simulink model "HEncoder"  (R2018b)
settings: Solver=VariableStepAuto  StartTime=0.0  StopTime=10.0  RelTol=1e-3
settings Model: Creator=bai  LastModifiedBy=bai

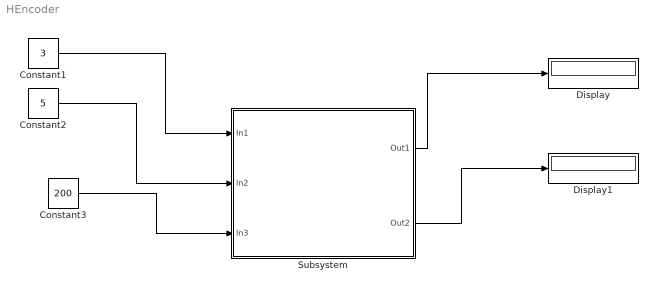
== system HEncoder ==
  Constant1 : Constant  Value=3
  Constant2 : Constant  Value=5
  Constant3 : Constant  Value=200
  Display : Display
  Display1 : Display
  Subsystem : Subsystem
      mask Display:
      | image('halleffect.jpg');
      | port_label('input', 1, 'A');
      | port_label('input', 2, 'B');
      | port_label('input', 3, 'sampleTIME');
      | port_label('output', 1, 'counter');
      | port_label('output', 2, 'rpm');
  wires:
  Constant1/1 -> Subsystem/1(In1)
  Constant2/1 -> Subsystem/2(In2)
  Constant3/1 -> Subsystem/3(In3)
  Subsystem/1(Out1) -> Display/1
  Subsystem/2(Out2) -> Display1/1

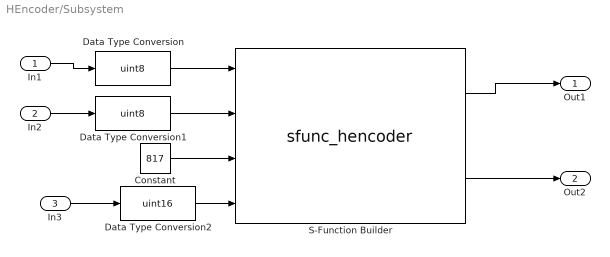
== system HEncoder/Subsystem ==
  In1 : Inport
  In2 : Inport  Port=2
  In3 : Inport  Port=3
  Constant : Constant  Value=817  OutDataTypeStr=uint16
  Data Type Conversion : DataTypeConversion  OutDataTypeStr=uint8
  Data Type Conversion1 : DataTypeConversion  OutDataTypeStr=uint8
  Data Type Conversion2 : DataTypeConversion  OutDataTypeStr=uint16
  S-Function Builder : S-Function  InitFcn=try, set_param(gcb,'FunctionName','sfunc_hencoder'), end  FunctionName=sfunc_hencoder  SFunctionModules=sfunc_hencoder_wrapper  SFunctionDeploymentMode=off  EnableBusSupport=off  mask(S-Function Builder){}
      mask help: Simulink:masks:SFunctionBuilder_MD
      mask init:
      | val = [[.9  0.75 0.75 1 1 .9 .9 1]',[1 1 0.75 0.75 .9 .9 1 .9]'];try , sys = get_param(gcb,'SfunBuilderFcnName');if isempty(sys), sys = get_param(gcb,'FunctionName'); end,catch, sys = get_param(gcb,'FunctionName'); end
      settings: CopyFcn=set_param(gcbh,'LinkStatus','none')  PreSaveFcn=try, set_param(gcb,'FunctionName','sfunc_hencoder'), end  OpenFcn=sfunctionwizard(gcbh)
      mask Display: plot(val(:,1),val(:,2)),disp(sys), port_label('input',1,'pinA'), port_label('input',2,'pinB'), port_label('input',3,'cntperrot'), port_label('input',4,'sampletime'), port_label('output',1,'pos'), port_label('output',2,'rpm')
  Out1 : Outport
  Out2 : Outport  Port=2
  wires:
  S-Function Builder/2 -> Out2/1
  S-Function Builder/1 -> Out1/1
  Constant/1 -> S-Function Builder/3
  Data Type Conversion/1 -> S-Function Builder/1
  In1/1 -> Data Type Conversion/1
  Data Type Conversion1/1 -> S-Function Builder/2
  In2/1 -> Data Type Conversion1/1
  Data Type Conversion2/1 -> S-Function Builder/4
  In3/1 -> Data Type Conversion2/1
